simulink model "simulareRST510"  (R2020a)
settings: Solver=ode4  StartTime=0.0  StopTime=200  RelTol=1e-3
settings Model: Creator=user  LastModifiedBy=user

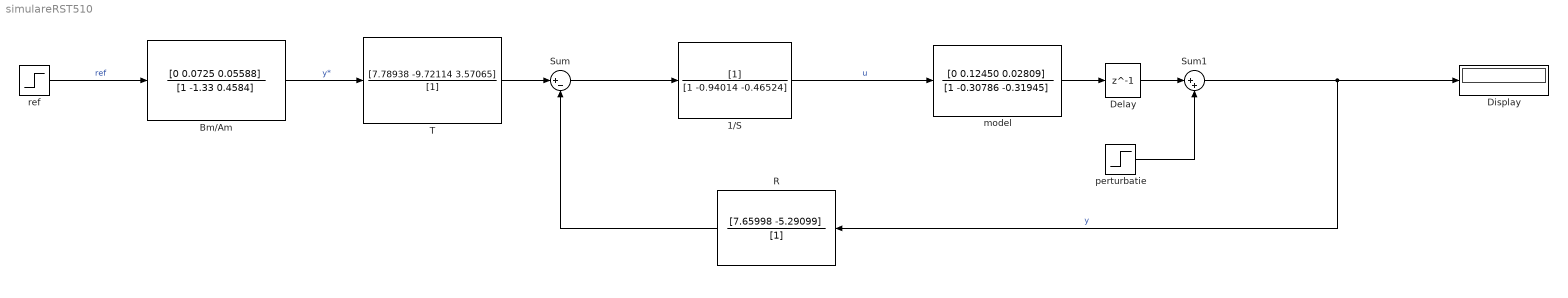
== system simulareRST510 ==
  1/S : DiscreteFilter  Denominator=[1 -0.94014 -0.46524]  SampleTime=0.6
  Bm/Am : DiscreteFilter  Numerator=[0 0.0725 0.05588]  Denominator=[1 -1.33 0.4584]  SampleTime=0.6
  Delay : Delay  DelayLength=1  SampleTime=0.6
  Display : Display
  R : DiscreteFilter  Numerator=[7.65998 -5.29099]  Denominator=[1]  SampleTime=0.6
  Sum : Sum  Inputs=|+-
  Sum1 : Sum  Inputs=|++
  T : DiscreteFilter  Numerator=[7.78938 -9.72114 3.57065]  Denominator=[1]  SampleTime=0.6
  model : DiscreteFilter  Numerator=[0 0.12450 0.02809]  Denominator=[1 -0.30786 -0.31945]  SampleTime=0.6
  perturbatie : Step  Time=50  After=0.25  SampleTime=0.6
  ref : Step  SampleTime=0.6
  wires:
  ref/1 -> Bm/Am/1  "ref"
  T/1 -> Sum/1
  Bm/Am/1 -> T/1  "y*"
  Sum/1 -> 1/S/1
  1/S/1 -> model/1  "u"
  R/1 -> Sum/2
  model/1 -> Delay/1
  perturbatie/1 -> Sum1/2
  Sum1/1 -> R/1, Display/1  "y"
  Delay/1 -> Sum1/1
